simulink model "GlwLmp_DD"  (R2016b)
settings: configuration reference "CodeGenConfigSet" (kept outside this file)
values from neighbouring files (symbols this model uses):
  GlwLmp_stPsDiaDisbl_C = Calibration.Parameter    [init_GlwLmp_DD.m]
  GlwLmp_stPsDisbl_C = Calibration.Parameter    [init_GlwLmp_DD.m]
  SigTst_stGlwLmp_C = Calibration.Parameter    [init_GlwLmp_DD.m]
  SigTst_swtGlwLmp_C = Calibration.Parameter    [init_GlwLmp_DD.m]
undefined symbols (not defined in the file or in its folder): Switch_conv
libraries: simulink x4
settings Model: Creator=lenovo  LastModifiedBy=liutao
settings ConfigSetRef: SourceLocation=Base Workspace

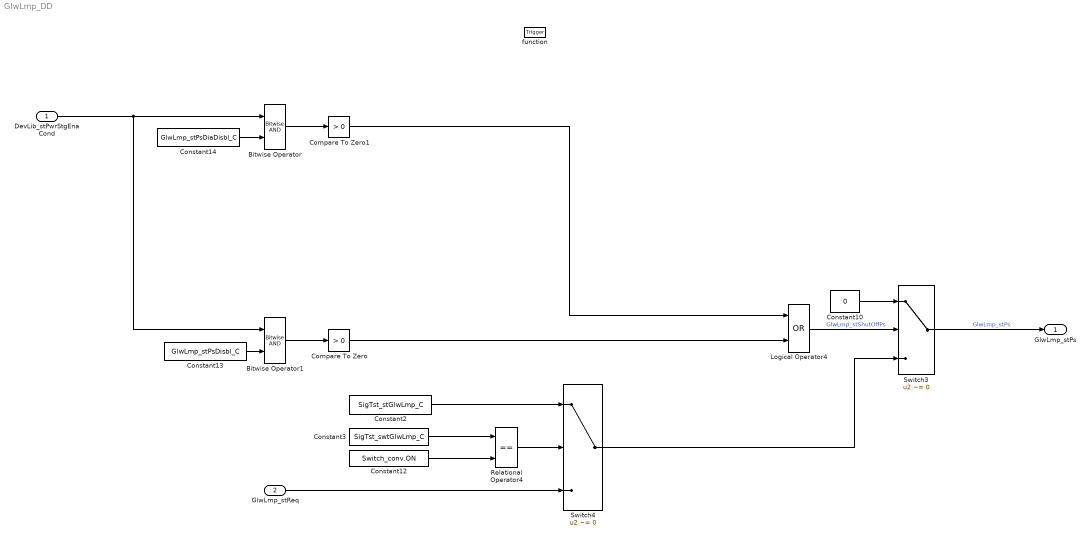
== system GlwLmp_DD ==
  DevLib_stPwrStgEnaCond : Inport  Description=Control unit status relevant to power stage deactivation/error diagnosis  OutMin=0  OutMax=65535  OutDataTypeStr=State_uint16
  GlwLmp_stReq : Inport  Description=Glow lamp request status  Port=2  OutMin=0  OutMax=1  OutDataTypeStr=boolean
  function : TriggerPort  TriggerType=function-call  VariantControl=Variant
  Bitwise Operator : simulink/Logic and Bit Operations/Bitwise Operator  logicop=AND  UseBitMask=off  NumInputPorts=2  BitMask=bin2dec('11011001')  BitMaskRealWorld=Stored Integer
  Bitwise Operator1 : simulink/Logic and Bit Operations/Bitwise Operator  logicop=AND  UseBitMask=off  NumInputPorts=2  BitMask=bin2dec('11011001')  BitMaskRealWorld=Stored Integer
  Compare To Zero : simulink/Logic and Bit Operations/Compare To Zero  relop=>  OutDataTypeStr=boolean
  Compare To Zero1 : simulink/Logic and Bit Operations/Compare To Zero  relop=>  OutDataTypeStr=uint8
  Constant10 : Constant  Value=0  OutDataTypeStr=boolean  SampleTime=-1
  Constant12 : Constant  Value=Switch_conv.ON
  Constant13 : Constant  Value=GlwLmp_stPsDisbl_C
  Constant14 : Constant  Value=GlwLmp_stPsDiaDisbl_C
  Constant2 : Constant  Value=SigTst_stGlwLmp_C
  Constant3 : Constant  Value=SigTst_swtGlwLmp_C
  Logical Operator4 : Logic  Operator=OR  AllPortsSameDT=off  OutDataTypeStr=boolean
  Relational Operator4 : RelationalOperator  Operator===  OutDataTypeStr=boolean  RndMeth=Nearest
  Switch3 : Switch  Criteria=u2 ~= 0  SaturateOnIntegerOverflow=on  InputSameDT=on
  Switch4 : Switch  Criteria=u2 ~= 0  SaturateOnIntegerOverflow=on  InputSameDT=on
  GlwLmp_stPs : Outport  Description=Digital output to the actuator after diagnosis  OutMin=0  OutMax=1  OutDataTypeStr=boolean
  wires:
  Bitwise Operator/1 -> Compare To Zero1/1
  Constant13/1 -> Bitwise Operator1/2
  Constant14/1 -> Bitwise Operator/2
  GlwLmp_stReq/1 -> Switch4/3
  Constant2/1 -> Switch4/1
  Relational Operator4/1 -> Switch4/2
  Constant3/1 -> Relational Operator4/1
  Constant12/1 -> Relational Operator4/2
  Compare To Zero/1 -> Logical Operator4/2
  Logical Operator4/1 -> Switch3/2  "GlwLmp_stShutOffPs"
  Switch4/1 -> Switch3/3
  Bitwise Operator1/1 -> Compare To Zero/1
  DevLib_stPwrStgEnaCond/1 -> Bitwise Operator/1, Bitwise Operator1/1
  Constant10/1 -> Switch3/1
  Switch3/1 -> GlwLmp_stPs/1  "GlwLmp_stPs"
  Compare To Zero1/1 -> Logical Operator4/1
